simulink model "Full_Dynamics_Model"  (R2024a)
settings: Solver=VariableStepAuto  StartTime=0.0  StopTime=10.0  RelTol=1e-3
undefined symbols (not defined in the file): F, g, Lambda, nu_b_0, Omega_r_0, p_b_i_0, q_0, T_max, T_min, T_trim, UAV
settings Model: Creator=Usuario  LastModifiedBy=Usuario

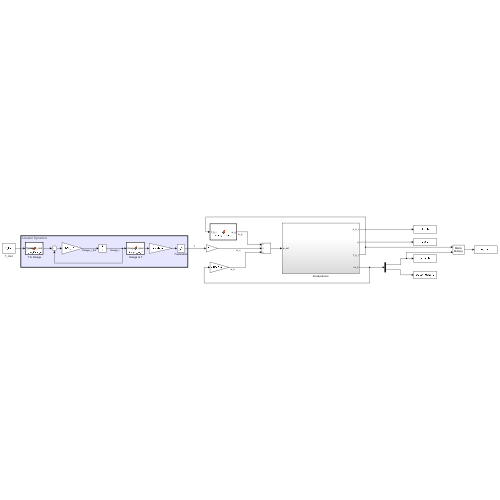
[thumbnail: Simulink's stored preview of the top-level diagram]
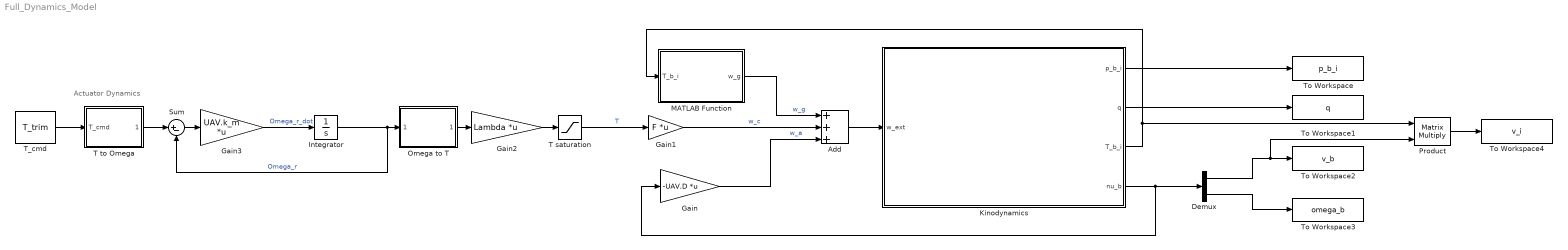
== system Full_Dynamics_Model ==
  note: Actuator Dynamics
  " Omega to T" : MATLAB Function  TreatAsAtomicUnit=on
  " T to Omega" : MATLAB Function  TreatAsAtomicUnit=on
  Add : Sum  Inputs=+++
  Demux : Demux  Outputs=[3 3]
  Gain : Gain  Gain=-UAV.D  Multiplication=Matrix(K*u)
  Gain1 : Gain  Gain=F  Multiplication=Matrix(K*u)
  Gain2 : Gain  Gain=Lambda  Multiplication=Matrix(K*u)
  Gain3 : Gain  Gain=UAV.k_m  Multiplication=Matrix(K*u)
  Integrator : Integrator  InitialCondition=Omega_r_0
  Kinodynamics : Subsystem
  MATLAB Function : MATLAB Function  TreatAsAtomicUnit=on
  Product : Product  Multiplication=Matrix(*)
  Sum : Sum  Inputs=|+-
  T saturation : Saturate  UpperLimit=T_max  LowerLimit=T_min
  T_cmd : Constant  Value=T_trim
  To Workspace : ToWorkspace  VariableName=p_b_i  SaveFormat=Timeseries  SampleTime=-1
  To Workspace1 : ToWorkspace  VariableName=q  SaveFormat=Timeseries  SampleTime=-1
  To Workspace2 : ToWorkspace  VariableName=v_b  SaveFormat=Timeseries  SampleTime=-1
  To Workspace3 : ToWorkspace  VariableName=omega_b  SaveFormat=Timeseries  SampleTime=-1
  To Workspace4 : ToWorkspace  VariableName=v_i  SaveFormat=Timeseries  SampleTime=-1
  wires:
  Kinodynamics/1(p_b_i) -> To Workspace/1
  Add/1 -> Kinodynamics/1(w_ext)
  Kinodynamics/2(q) -> To Workspace1/1
  Kinodynamics/3(T_b_i) -> MATLAB Function/1(T_b_i), Product/1
  Demux/2 -> To Workspace3/1
  MATLAB Function/1(w_g) -> Add/1  "w_g"
  Demux/1 -> Product/2, To Workspace2/1
  Gain/1 -> Add/3  "w_a"
  Kinodynamics/4(nu_b) -> Gain/1, Demux/1
  Gain1/1 -> Add/2  "w_c"
  T_cmd/1 -> " T to Omega"/1(T_cmd)
  " Omega to T"/1(T_ideal) -> Gain2/1
  " T to Omega"/1(Omega_r_cmd) -> Sum/1
  Sum/1 -> Gain3/1
  T saturation/1 -> Gain1/1  "T"
  Integrator/1 -> " Omega to T"/1(Omega_r), Sum/2  "Omega_r"
  Gain3/1 -> Integrator/1  "Omega_r_dot"
  Gain2/1 -> T saturation/1
  Product/1 -> To Workspace4/1

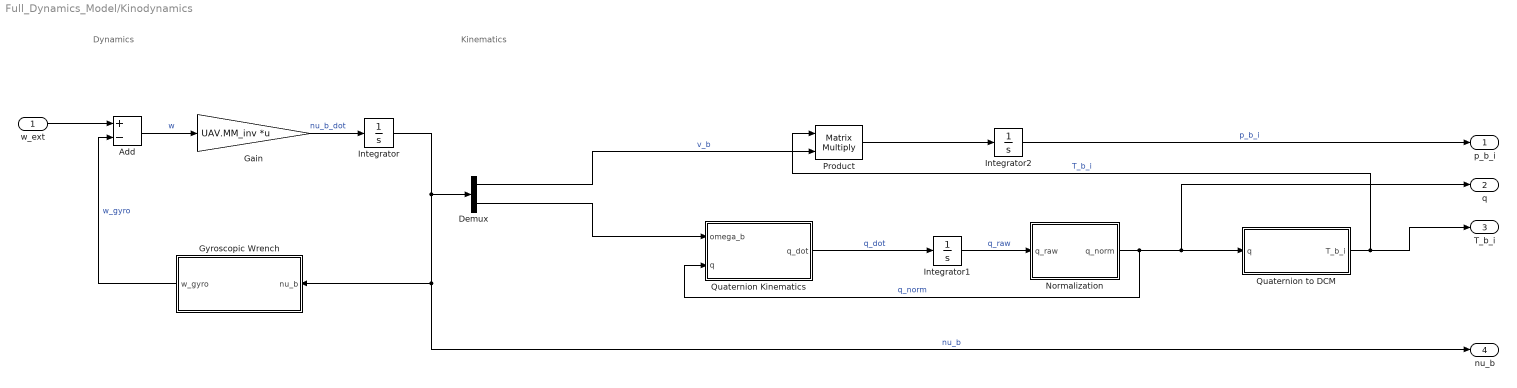
== system Full_Dynamics_Model/Kinodynamics ==
  note: Dynamics
  note: Kinematics
  w_ext : Inport
  " Normalization" : MATLAB Function  TreatAsAtomicUnit=on
  Add : Sum  Inputs=+-
  Demux : Demux  Outputs=[3 3]
  Gain : Gain  Gain=UAV.MM_inv  Multiplication=Matrix(K*u)
  Gyroscopic Wrench : MATLAB Function  TreatAsAtomicUnit=on
  Integrator : Integrator  InitialCondition=nu_b_0
  Integrator1 : Integrator  InitialCondition=q_0
  Integrator2 : Integrator  InitialCondition=p_b_i_0
  Product : Product  Multiplication=Matrix(*)
  Quaternion Kinematics : MATLAB Function  TreatAsAtomicUnit=on
  Quaternion to DCM : MATLAB Function  TreatAsAtomicUnit=on
  p_b_i : Outport
  q : Outport  Port=2
  T_b_i : Outport  Port=3
  nu_b : Outport  Port=4
  wires:
  Integrator2/1 -> p_b_i/1  "p_b_i"
  Demux/1 -> Product/2  "v_b"
  Quaternion to DCM/1(T_b_i) -> T_b_i/1, Product/1  "T_b_i"
  Product/1 -> Integrator2/1
  Quaternion Kinematics/1(q_dot) -> Integrator1/1  "q_dot"
  Demux/2 -> Quaternion Kinematics/1(omega_b)
  " Normalization"/1(q_norm) -> q/1, Quaternion to DCM/1(q), Quaternion Kinematics/2(q)  "q_norm"
  Integrator1/1 -> " Normalization"/1(q_raw)  "q_raw"
  Gain/1 -> Integrator/1  "nu_b_dot"
  w_ext/1 -> Add/1
  Add/1 -> Gain/1  "w"
  Gyroscopic Wrench/1(w_gyro) -> Add/2  "w_gyro"
  Integrator/1 -> Demux/1, nu_b/1, Gyroscopic Wrench/1(nu_b)  "nu_b"

== matlab function Full_Dynamics_Model/Kinodynamics/ Normalization ==
  data: q_raw input; q_norm output
function q_norm=normalization(q_raw)

q_norm=q_raw/norm(q_raw);

== matlab function Full_Dynamics_Model/Kinodynamics/Quaternion Kinematics ==
  data: omega_b input; q_dot output; q input
function q_dot = quat_kinematics(omega_b,q)
%Quaternion kinematics. Requires that omega_b be a column vector. q must
%also be a column vector following the course's quaternion convention. 
eta=q(1);
epsilon=q(2:4);
epsilon_x=cross_matrix(epsilon);

q_dot=1/2*[-epsilon';epsilon_x+eta*eye(3,3)]*omega_b;
end

== matlab function Full_Dynamics_Model/Kinodynamics/Gyroscopic Wrench ==
  data: nu_b input; w_gyro output; UAV parameter
function w_gyro=gyroscopic_wrench(nu_b,UAV)
nu_b_southwest=[cross_matrix(nu_b(4:6)),zeros(3,3);cross_matrix(nu_b(1:3)),cross_matrix(nu_b(4:6))];
w_gyro=nu_b_southwest*UAV.MM*nu_b;
end

== matlab function Full_Dynamics_Model/MATLAB Function ==
  data: T_b_i input; w_g output; UAV parameter; g parameter
function w_g=Gravity_Wrench(T_b_i,UAV, g)
e3=[0;0;1];

w_g=-g*[UAV.m*T_b_i'*e3;UAV.S*T_b_i'*e3];
end

== matlab function Full_Dynamics_Model/ T to Omega ==
  data: T_cmd input; Omega_r_cmd output; k_f parameter
function Omega_r_cmd=T_to_Omega(T_cmd,k_f)
Omega_r_cmd=sqrt(T_cmd/k_f);
end

== matlab function Full_Dynamics_Model/ Omega to T ==
  data: Omega_r input; T_ideal output; k_f parameter
function T_ideal=Omega_to_T(Omega_r,k_f)
T_ideal=k_f*Omega_r.^2;
end

== matlab function Full_Dynamics_Model/Kinodynamics/Quaternion to DCM ==
  data: q input; T_b_i output
function T_b_i=quaternion_to_DCM(q)
%My implementation of the quaternion to DCM transformation, to ensure
%consistency. It must return the active representation of the rotation
%between i and b, which will be the DCM from b to i. 
eta=q(1);
epsilon=q(2:4);
epsilon_x=cross_matrix(epsilon);

T_b_i=eye(3,3)+2*eta*epsilon_x+2*epsilon_x*epsilon_x;
end
